simulink model "vehicle_hardware"  (Simulink 7.7)
settings: Solver=ode45  StartTime=0.0  StopTime=10.0  RelTol=1e-3
undefined symbols (not defined in the file): num_robots
libraries: UAVdesign_net x20
settings Model: Creator=Emanuel  LastModifiedBy=Emanuel
settings DebuggingCC: StrictBusMsg=Warning
settings SFSimCC: SimParseCustomCode=off

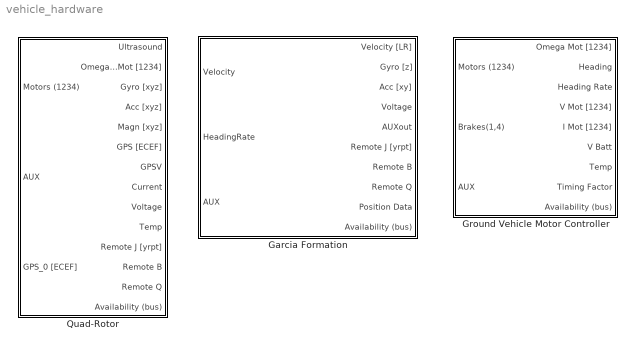
== system vehicle_hardware ==
  Garcia Formation : Subsystem  mask(GarciaFormation){robots_list=[0 1 2 3], sensors_list=[0 1 2 3], use_sensors=off, devicetype=UDP port, com_port='COM4', baud=115200, host_name='192.168.1.10', remote_port=60500, local_port=60500, timeout=1, sample_time=1/20}
      mask prompts: robots_list "List of robots"; sensors_list "List of ultrasound+radio sensors"; use_sensors "Use ultrasound sensors"; devicetype "Device Type"; com_port "COM port (string between commas, e.g. 'COM4')"; baud "Baud Rate"; host_name "Host Name (string between commas, e.g. '192.168.1.10')"; remote_port "Remote UDP port"; local_port "Local UDP port"; timeout "Timeout (sec)"; sample_time "Sample Time"
      mask help:
      | Hardware interface for the Garcia & Track robot formation.
      |
      | If Timeout is zero, the block will not delay the simulation until the data packets arrive. If Timeout is positive and no packet arrives until it elapses, an error will be generated and the simulation will stop.
      mask init:
      | start = 3;
      | a=get_param([gcb '/Generic Comm'], 'MaskStyles');
      | b=get_param(gcb, 'MaskStyles');
      | b{start+1}=a{1};
      | set_param(gcb, 'MaskStyles', b);
      | 
      | a=get_param(gcb, 'MaskValues');
      | b=get_param([gcb '/Generic Comm'], 'MaskValues');
      | b{1}=a{start+1};
      | set_param([gcb '/Generic Comm'], 'MaskValues', b);
      mask StyleString: edit,edit,checkbox,popup(COM port|UDP port),edit,edit,edit,edit,edit,edit,edit
      mask CallbackString:
      | |||start = 3;
      | UAVdesign_net_generic_comm_callback(gcb, 1, start)|||||||
      mask Display:
      | text(0.1, 0.30, ['sensors: ' num2str(sensors_list)])
      | text(0.1, 0.40, ['robots: ' num2str(robots_list)])
      | text(0.1, 0.70, com_port)
      | text(0.1, 0.60, host_name)
  Ground Vehicle Motor Controller : Subsystem  mask(GroundVehicle){com_port='COM4', timeout=1, sample_time=1/100}
      mask prompts: com_port "COM port"; timeout "Timeout (sec)"; sample_time "Sample Time"
      mask help:
      | Hardware interface for the Ground Vehicle Motor Controller.
      |
      | COM port has to be a string including commas, e.g. 'COM4'.
      | If Timeout is zero, the block will not delay the simulation until the data packets arrive. If Timeout is positive and no packet arrives until it elapses, an error will be generated and the simulation will stop.
      mask Display: disp(com_port)
  Quad-Rotor : Subsystem  mask(QuadRotor){devicetype=UDP port, com_port='COM4', baud=115200, host_name='192.168.1.10', remote_port=60500, local_port=60500, timeout=1, sample_time=1/50}
      mask prompts: devicetype "Device Type"; com_port "COM port (string between commas, e.g. 'COM4')"; baud "Baud Rate"; host_name "Host Name (string between commas, e.g. '192.168.1.10')"; remote_port "Remote UDP port"; local_port "Local UDP port"; timeout "Timeout (sec)"; sample_time "Sample Time"
      mask help:
      | Hardware interface for the QuadRotor.
      |
      | COM port has to be a string including commas, e.g. 'COM4'.
      | If Timeout is zero, the block will not delay the simulation until the data packets arrive. If Timeout is positive and no packet arrives until it elapses, an error will be generated and the simulation will stop.
      mask init:
      | start = 0;
      | a=get_param([gcb '/Generic Comm'], 'MaskStyles');
      | b=get_param(gcb, 'MaskStyles');
      | b{start+1}=a{1};
      | set_param(gcb, 'MaskStyles', b);
      | 
      | a=get_param(gcb, 'MaskValues');
      | b=get_param([gcb '/Generic Comm'], 'MaskValues');
      | b{1}=a{start+1};
      | set_param([gcb '/Generic Comm'], 'MaskValues', b);
      mask StyleString: popup(COM port|UDP port),edit,edit,edit,edit,edit,edit,edit
      mask CallbackString:
      | start = 0;
      | UAVdesign_net_generic_comm_callback(gcb, 1, start)|||||||
      mask Display: disp([com_port '\n' host_name])

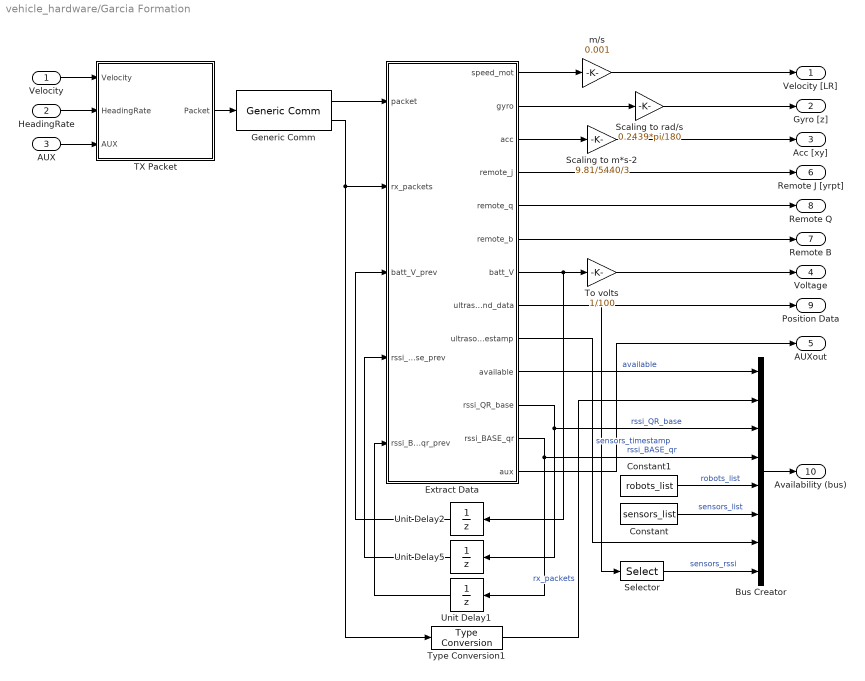
== system vehicle_hardware/Garcia Formation ==
  Velocity : Inport
  HeadingRate : Inport  Port=2
  AUX : Inport  Port=3
  Bus Creator : BusCreator  Inputs=8
  Constant : Constant  Value=sensors_list
  Constant1 : Constant  Value=robots_list
  Extract Data : Stateflow chart  TreatAsAtomicUnit=on
  Generic Comm : UAVdesign_net/Hardware/Generic Comm  SystemSampleTime=-1  devicetype=UDP port  com_port=com_port  baud=baud  host_name=host_name  remote_port=remote_port  local_port=local_port  timeout=timeout  rx_size=(max(robots_list)+1) * 16 + 18 + (4 + 17*8)*use_sensors  handshake=on  sample_time=sample_time
  Scaling to m*s-2 : Gain  Gain=9.81/5440/3
  Scaling to rad/s : Gain  Gain=0.2439*pi/180
  Selector : Selector  InputPortWidth=9*length(sensors_list)*use_sensors + (1-use_sensors)*1  IndexOptions=Index vector (dialog)  Indices=[9*(0:(length(sensors_list)-1)*use_sensors)+9*use_sensors+(1-use_sensors)]  OutputSizes=1
  TX Packet : Subsystem  TreatAsAtomicUnit=on
  To volts : Gain  Gain=1/100
  Type Conversion1 : UAVdesign_net/Hardware/Type Conversion  indim=1  intype=uint32  outdim=1  outtype=double  signextend=off
  Unit Delay1 : UnitDelay  X0=-100*ones(length(robots_list), 1)  SampleTime=-1
  Unit Delay2 : UnitDelay  X0=zeros(length(robots_list), 1)  SampleTime=-1
  Unit Delay5 : UnitDelay  X0=-100*ones(length(robots_list), 1)  SampleTime=-1
  m/s : Gain  Gain=0.001
  Velocity [LR] : Outport
  Gyro [z] : Outport  Port=2
  Acc [xy] : Outport  Port=3
  Voltage : Outport  Port=4
  AUXout : Outport  Port=5
  Remote J [yrpt] : Outport  Port=6
  Remote B : Outport  Port=7
  Remote Q : Outport  Port=8
  Position Data : Outport  Port=9
  Availability (bus) : Outport  Port=10
  wires:
  Extract Data/13(aux) -> AUXout/1
  AUX/1 -> TX Packet/3(AUX)
  Selector/1 -> Bus Creator/8  "sensors_rssi"
  Extract Data/8(ultrasound_data) -> Selector/1, Position Data/1
  Extract Data/9(ultrasound_timestamp) -> Bus Creator/7  "sensors_timestamp"
  Constant/1 -> Bus Creator/6  "sensors_list"
  Constant1/1 -> Bus Creator/5  "robots_list"
  Type Conversion1/1 -> Bus Creator/2  "rx_packets"
  Unit Delay1/1 -> Extract Data/5(rssi_BASE_qr_prev)
  Extract Data/12(rssi_BASE_qr) -> Bus Creator/4, Unit Delay1/1  "rssi_BASE_qr"
  Extract Data/5(remote_q) -> Remote Q/1
  Unit Delay5/1 -> Extract Data/4(rssi_QR_base_prev)
  Extract Data/11(rssi_QR_base) -> Bus Creator/3, Unit Delay5/1  "rssi_QR_base"
  Generic Comm/2 -> Type Conversion1/1, Extract Data/2(rx_packets)
  Unit Delay2/1 -> Extract Data/3(batt_V_prev)
  Generic Comm/1 -> Extract Data/1(packet)
  Extract Data/10(available) -> Bus Creator/1  "available"
  Extract Data/7(batt_V) -> To volts/1, Unit Delay2/1
  Extract Data/6(remote_b) -> Remote B/1
  Extract Data/4(remote_j) -> Remote J [yrpt]/1
  Extract Data/3(acc) -> Scaling to m*s-2/1
  Extract Data/2(gyro) -> Scaling to rad/s/1
  Extract Data/1(speed_mot) -> m/s/1
  Scaling to m*s-2/1 -> Acc [xy]/1
  Scaling to rad/s/1 -> Gyro [z]/1
  m/s/1 -> Velocity [LR]/1
  Bus Creator/1 -> Availability (bus)/1
  To volts/1 -> Voltage/1
  Velocity/1 -> TX Packet/1(Velocity)
  TX Packet/1(Packet) -> Generic Comm/1
  HeadingRate/1 -> TX Packet/2(HeadingRate)

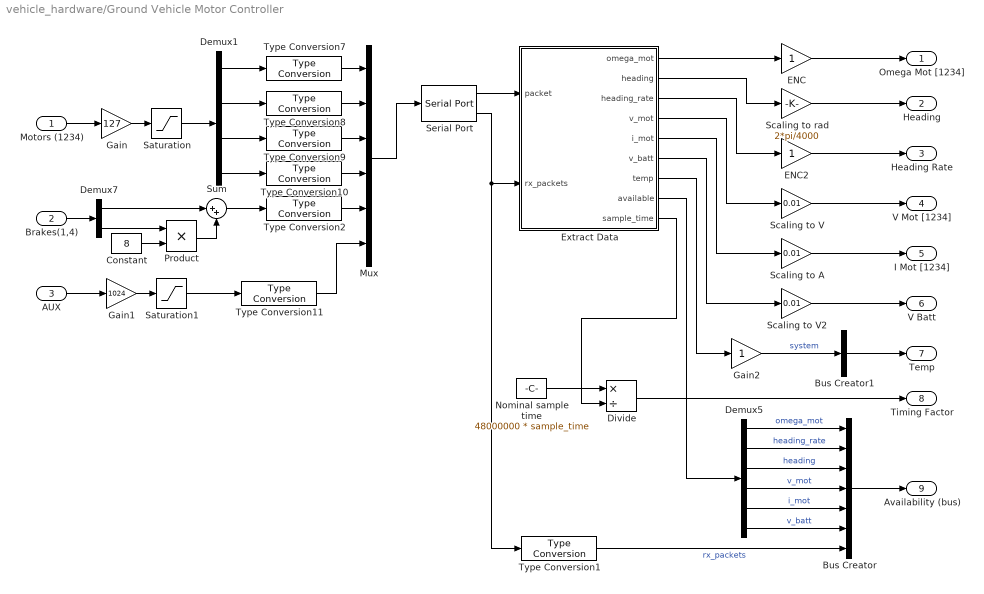
== system vehicle_hardware/Ground Vehicle Motor Controller ==
  Motors (1234) : Inport
  Brakes(1,4) : Inport  Port=2  OutDataTypeStr=boolean  PortDimensions=2
  AUX : Inport  Port=3
  Bus Creator : BusCreator  Inputs=7
  Bus Creator1 : BusCreator  Inputs=1
  Constant : Constant  Value=8
  Demux1 : Demux
  Demux5 : Demux  Outputs=[4 1 1 4 4 1]
  Demux7 : Demux  Outputs=2
  Divide : Product  Inputs=*/
  ENC : Gain
  ENC2 : Gain
  Extract Data : Stateflow chart  TreatAsAtomicUnit=on
  Gain : Gain  Gain=127
  Gain1 : Gain  Gain=1024
  Gain2 : Gain
  Mux : Mux  Inputs=6
  Nominal sample time : Constant  Value=48000000 * sample_time
  Product : Product  RndMeth=Zero
  Saturation : Saturate  UpperLimit=127  LowerLimit=-127
  Saturation1 : Saturate  UpperLimit=1023  LowerLimit=0
  Scaling to A : Gain  Gain=0.01
  Scaling to V : Gain  Gain=0.01
  Scaling to V2 : Gain  Gain=0.01
  Scaling to rad : Gain  Gain=2*pi/4000
  Serial Port : UAVdesign_net/Hardware/Serial Port  port=com_port  baud_rate=115200  timeout=timeout  tx_enable=on  rx_enable=on  receive=56  num_packets_overrun=off  num_packets_received=on  st=sample_time
  Sum : Sum  Inputs=|++  OutDataTypeStr=uint16
  Type Conversion1 : UAVdesign_net/Hardware/Type Conversion  indim=1  intype=uint32  outdim=1  outtype=double  signextend=off
  Type Conversion{7..11} (5 alike) : UAVdesign_net/Hardware/Type Conversion  indim=1  intype=double  outdim=2  outtype=uint8  signextend=off
  Type Conversion2 : UAVdesign_net/Hardware/Type Conversion  indim=1  intype=uint16  outdim=2  outtype=uint8  signextend=off
  Omega Mot [1234] : Outport
  Heading : Outport  Port=2
  Heading Rate : Outport  Port=3
  V Mot [1234] : Outport  Port=4
  I Mot [1234] : Outport  Port=5
  V Batt : Outport  Port=6
  Temp : Outport  Port=7
  Timing Factor : Outport  Port=8
  Availability (bus) : Outport  Port=9
  wires:
  Type Conversion1/1 -> Bus Creator/7  "rx_packets"
  Serial Port/2 -> Extract Data/2(rx_packets), Type Conversion1/1
  Serial Port/1 -> Extract Data/1(packet)
  Extract Data/8(available) -> Demux5/1
  Scaling to V/1 -> V Mot [1234]/1
  Scaling to rad/1 -> Heading/1
  Bus Creator1/1 -> Temp/1
  Bus Creator/1 -> Availability (bus)/1
  Scaling to V2/1 -> V Batt/1
  Gain1/1 -> Saturation1/1
  Saturation1/1 -> Type Conversion11/1
  Saturation/1 -> Demux1/1
  Gain/1 -> Saturation/1
  Motors (1234)/1 -> Gain/1
  Scaling to A/1 -> I Mot [1234]/1
  Mux/1 -> Serial Port/1
  Type Conversion10/1 -> Mux/4
  Type Conversion9/1 -> Mux/3
  Type Conversion8/1 -> Mux/2
  Type Conversion7/1 -> Mux/1
  AUX/1 -> Gain1/1
  Demux1/1 -> Type Conversion7/1
  Demux1/2 -> Type Conversion8/1
  Demux1/3 -> Type Conversion9/1
  Demux1/4 -> Type Conversion10/1
  Brakes(1,4)/1 -> Demux7/1
  Demux7/2 -> Product/1
  Constant/1 -> Product/2
  Sum/1 -> Type Conversion2/1
  Demux7/1 -> Sum/1
  Product/1 -> Sum/2
  Type Conversion11/1 -> Mux/6
  Gain2/1 -> Bus Creator1/1  "system"
  Demux5/1 -> Bus Creator/1  "omega_mot"
  Extract Data/1(omega_mot) -> ENC/1
  Extract Data/2(heading) -> Scaling to rad/1
  Extract Data/4(v_mot) -> Scaling to V/1
  Extract Data/5(i_mot) -> Scaling to A/1
  Extract Data/6(v_batt) -> Scaling to V2/1
  Extract Data/7(temp) -> Gain2/1
  Type Conversion2/1 -> Mux/5
  Extract Data/9(sample_time) -> Divide/2
  Divide/1 -> Timing Factor/1
  Nominal sample time/1 -> Divide/1
  ENC/1 -> Omega Mot [1234]/1
  Demux5/6 -> Bus Creator/6  "v_batt"
  Demux5/5 -> Bus Creator/5  "i_mot"
  Demux5/4 -> Bus Creator/4  "v_mot"
  Demux5/3 -> Bus Creator/3  "heading"
  Demux5/2 -> Bus Creator/2  "heading_rate"
  ENC2/1 -> Heading Rate/1
  Extract Data/3(heading_rate) -> ENC2/1

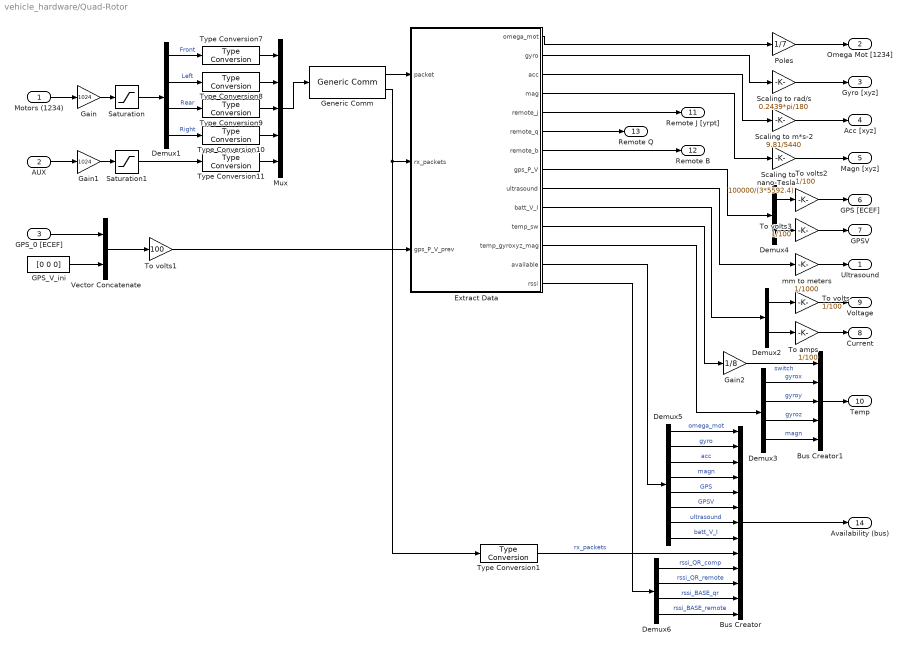
== system vehicle_hardware/Quad-Rotor ==
  Motors (1234) : Inport
  AUX : Inport  Port=2
  GPS_0 [ECEF] : Inport  Port=3
  Bus Creator : BusCreator  Inputs=13
  Bus Creator1 : BusCreator  Inputs=5
  Demux1 : Demux
  Demux2 : Demux  Outputs=2
  Demux3 : Demux
  Demux4 : Demux  Outputs=2
  Demux5 : Demux  Outputs=[4 3 3 3 3 3 1 1]
  Demux6 : Demux
  Extract Data : Stateflow chart  TreatAsAtomicUnit=on
  GPS_V_ini : Constant  Value=[0 0 0]
  Gain : Gain  Gain=1024
  Gain1 : Gain  Gain=1024
  Gain2 : Gain  Gain=1/8
  Generic Comm : UAVdesign_net/Hardware/Generic Comm  SystemSampleTime=-1  devicetype=UDP port  com_port=com_port  baud=baud  host_name=host_name  remote_port=remote_port  local_port=local_port  timeout=timeout  rx_size=54  handshake=on  sample_time=sample_time
  Mux : Mux  Inputs=5
  Poles : Gain  Gain=1/7
  Saturation : Saturate  UpperLimit=1023  LowerLimit=0
  Saturation1 : Saturate  UpperLimit=1023  LowerLimit=0
  Scaling to m*s-2 : Gain  Gain=9.81/5440
  Scaling to nano-Tesla : Gain  Gain=100000/(3*5592.4)
  Scaling to rad/s : Gain  Gain=0.2439*pi/180
  To amps : Gain  Gain=1/100
  To volts : Gain  Gain=1/100
  To volts1 : Gain  Gain=100
  To volts2 : Gain  Gain=1/100
  To volts3 : Gain  Gain=1/100
  Type Conversion1 : UAVdesign_net/Hardware/Type Conversion  indim=1  intype=uint32  outdim=1  outtype=double  signextend=off
  Type Conversion{7..11} (5 alike) : UAVdesign_net/Hardware/Type Conversion  indim=1  intype=double  outdim=2  outtype=uint8  signextend=off
  Vector Concatenate : Concatenate  Mode=Vector
  mm to meters : Gain  Gain=1/1000
  Ultrasound : Outport
  Omega Mot [1234] : Outport  Port=2
  Gyro [xyz] : Outport  Port=3
  Acc [xyz] : Outport  Port=4
  Magn [xyz] : Outport  Port=5
  GPS [ECEF] : Outport  Port=6
  GPSV : Outport  Port=7
  Current : Outport  Port=8
  Voltage : Outport  Port=9
  Temp : Outport  Port=10
  Remote J [yrpt] : Outport  Port=11
  Remote B : Outport  Port=12
  Remote Q : Outport  Port=13
  Availability (bus) : Outport  Port=14
  wires:
  Extract Data/6(remote_q) -> Remote Q/1
  Type Conversion1/1 -> Bus Creator/9  "rx_packets"
  Demux6/4 -> Bus Creator/13  "rssi_BASE_remote"
  Demux6/3 -> Bus Creator/12  "rssi_BASE_qr"
  Demux6/2 -> Bus Creator/11  "rssi_QR_remote"
  Demux6/1 -> Bus Creator/10  "rssi_QR_comp"
  Extract Data/14(rssi) -> Demux6/1
  Generic Comm/2 -> Type Conversion1/1, Extract Data/2(rx_packets)
  GPS_V_ini/1 -> Vector Concatenate/2
  GPS_0 [ECEF]/1 -> Vector Concatenate/1
  Vector Concatenate/1 -> To volts1/1
  To volts1/1 -> Extract Data/3(gps_P_V_prev)
  Generic Comm/1 -> Extract Data/1(packet)
  Extract Data/13(available) -> Demux5/1
  Demux5/8 -> Bus Creator/8  "batt_V_I"
  Demux5/7 -> Bus Creator/7  "ultrasound"
  Demux5/6 -> Bus Creator/6  "GPSV"
  Demux5/5 -> Bus Creator/5  "GPS"
  Demux5/4 -> Bus Creator/4  "magn"
  Demux5/3 -> Bus Creator/3  "acc"
  Demux5/2 -> Bus Creator/2  "gyro"
  Demux5/1 -> Bus Creator/1  "omega_mot"
  Extract Data/12(temp_gyroxyz_mag) -> Demux3/1
  Extract Data/11(temp_sw) -> Gain2/1
  Extract Data/10(batt_V_I) -> Demux2/1
  Extract Data/9(ultrasound) -> mm to meters/1
  Extract Data/7(remote_b) -> Remote B/1
  Extract Data/5(remote_j) -> Remote J [yrpt]/1
  Extract Data/4(mag) -> Scaling to nano-Tesla/1
  Extract Data/3(acc) -> Scaling to m*s-2/1
  Extract Data/2(gyro) -> Scaling to rad/s/1
  Extract Data/1(omega_mot) -> Poles/1
  Extract Data/8(gps_P_V) -> Demux4/1
  Demux4/2 -> To volts3/1
  Demux4/1 -> To volts2/1
  To volts3/1 -> GPSV/1
  To volts2/1 -> GPS [ECEF]/1
  Scaling to m*s-2/1 -> Acc [xyz]/1
  Scaling to rad/s/1 -> Gyro [xyz]/1
  Poles/1 -> Omega Mot [1234]/1
  Demux2/2 -> To amps/1
  Demux2/1 -> To volts/1
  Demux3/4 -> Bus Creator1/5  "magn"
  Demux3/3 -> Bus Creator1/4  "gyroz"
  Demux3/2 -> Bus Creator1/3  "gyroy"
  Demux3/1 -> Bus Creator1/2  "gyrox"
  Gain2/1 -> Bus Creator1/1  "switch"
  Bus Creator1/1 -> Temp/1
  Bus Creator/1 -> Availability (bus)/1
  To volts/1 -> Voltage/1
  To amps/1 -> Current/1
  mm to meters/1 -> Ultrasound/1
  Gain1/1 -> Saturation1/1
  Saturation1/1 -> Type Conversion11/1
  Saturation/1 -> Demux1/1
  Gain/1 -> Saturation/1
  Demux1/3 -> Type Conversion9/1  "Rear"
  Demux1/2 -> Type Conversion8/1  "Left"
  Demux1/4 -> Type Conversion10/1  "Right"
  Demux1/1 -> Type Conversion7/1  "Front"
  Motors (1234)/1 -> Gain/1
  Scaling to nano-Tesla/1 -> Magn [xyz]/1
  Mux/1 -> Generic Comm/1
  Type Conversion11/1 -> Mux/5
  Type Conversion10/1 -> Mux/4
  Type Conversion9/1 -> Mux/3
  Type Conversion8/1 -> Mux/2
  Type Conversion7/1 -> Mux/1
  AUX/1 -> Gain1/1

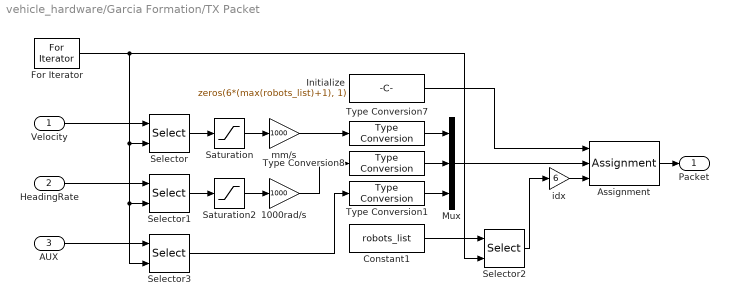
== system vehicle_hardware/Garcia Formation/TX Packet ==
  Velocity : Inport
  HeadingRate : Inport  Port=2
  AUX : Inport  Port=3  OutDataTypeStr=uint16
  1000rad/s : Gain  Gain=1000
  Assignment : Assignment  IndexMode=Zero-based  IndexOptions=Starting index (port)  Indices=1  OutputSizes=num_robots * 4
  Constant1 : Constant  Value=robots_list  OutDataTypeStr=uint32
  For Iterator : ForIterator  IterationLimit=length(robots_list)  IndexMode=Zero-based
  Initialize : Constant  Value=zeros(6*(max(robots_list)+1), 1)  OutDataTypeStr=uint8
  Mux : Mux  Inputs=3
  Saturation : Saturate  UpperLimit=1  LowerLimit=-1
  Saturation2 : Saturate  UpperLimit=2*pi  LowerLimit=-2*pi
  Selector{,1..3} (4 alike) : Selector  IndexMode=Zero-based  InputPortWidth=length(robots_list)  IndexOptions=Starting index (port)  Indices=[1 3]  OutputSizes=1
  Type Conversion1 : UAVdesign_net/Hardware/Type Conversion  indim=1  intype=uint16  outdim=2  outtype=uint8  signextend=off
  Type Conversion7 : UAVdesign_net/Hardware/Type Conversion  indim=1  intype=double  outdim=2  outtype=uint8  signextend=off
  Type Conversion8 : UAVdesign_net/Hardware/Type Conversion  indim=1  intype=double  outdim=2  outtype=uint8  signextend=off
  idx : Gain  Gain=6  ParamDataTypeStr=int32  OutDataTypeStr=int32
  mm/s : Gain  Gain=1000
  Packet : Outport
  wires:
  Type Conversion1/1 -> Mux/3
  Selector3/1 -> Type Conversion1/1
  AUX/1 -> Selector3/1
  Selector2/1 -> idx/1
  idx/1 -> Assignment/3
  Constant1/1 -> Selector2/1
  Initialize/1 -> Assignment/1
  Mux/1 -> Assignment/2
  Assignment/1 -> Packet/1
  For Iterator/1 -> Selector2/2, Selector3/2, Selector1/2, Selector/2
  HeadingRate/1 -> Selector1/1
  Selector1/1 -> Saturation2/1
  Selector/1 -> Saturation/1
  Velocity/1 -> Selector/1
  Type Conversion8/1 -> Mux/2
  Type Conversion7/1 -> Mux/1
  Saturation/1 -> mm/s/1
  Saturation2/1 -> 1000rad/s/1
  mm/s/1 -> Type Conversion7/1
  1000rad/s/1 -> Type Conversion8/1

== matlab function Garcia Formation/Extract Data ==
  data: packet input uint8; rx_packets input uint32; speed_mot output double; gyro output double; acc output double; remote_j output double size=4; remote_q output double size=4; remote_b output uint16 size=1; batt_V output double; ultrasound_data output double; ultrasound_timestamp output double; available output boolean; batt_V_prev input double; rssi_QR_base output double; rssi_QR_base_prev input double; robots_list parameter double; rssi_BASE_qr_prev input double; rssi_BASE_qr output double; sensors_list parameter double; use_sensors parameter double; aux output uint8
function [speed_mot,gyro, acc, remote_j, remote_q, remote_b, batt_V, ultrasound_data, ultrasound_timestamp, available, rssi_QR_base, rssi_BASE_qr, aux] = unpack(packet, rx_packets, batt_V_prev, rssi_QR_base_prev, robots_list, rssi_BASE_qr_prev, sensors_list, use_sensors)

robot_packet_size = 16;
num_robots = length(robots_list);
if num_robots < 1 || num_robots > 8
    error('A mimimum of 1 and a maximum of 8 robots can be used.');
end
if min(robots_list) < 0 || max(robots_list) > 7
   error('The robot identifiers must be between 0 and 7.'); 
end

speed_mot =         zeros(2*num_robots, 1);
gyro      =         zeros(  num_robots, 1);
acc       =         zeros(2*num_robots, 1);
aux       =         zeros(num_robots, 1, 'uint8');
available = logical(zeros(  num_robots, 1));

batt_V       = batt_V_prev;
rssi_QR_base = rssi_QR_base_prev;
rssi_BASE_qr = rssi_BASE_qr_prev;

for i=1:num_robots
    
    start = robots_list(i)*robot_packet_size;       % start of packet for the current robot (zero based)
    
    if rx_packets > 0
        MUX = uint8(packet(start+10));
    else
        MUX = uint8(0);
    end

    if MUX
        available(i) = logical(1);
    else
        available(i) = logical(0);
        rssi_QR_base(i) = -100;
        rssi_BASE_qr(i) = -100;
    end

    switch MUX
        case 4
            batt_V(i) = double(typecast(packet(start+(7:8)), 'uint16'));
        case 8
            rssi_QR_base(i) = -double(typecast(packet(start+5), 'uint8'));
            rssi_BASE_qr(i) = -double(typecast(packet(start+7), 'uint8'));
    end

    % speed_mot is actually the linear velocity in mm/sec for each wheel
    speed_mot(2*(i-1)+(1:2)) = double(typecast(packet(start+(11:14)), 'int16'));

    % the gyroscope data has to be scaled externally to rad/sec
    gyro(i) = double(typecast(packet(start+(15:16)), 'int16'));

    % the acceleration data has to be scaled externally to m/sec^2
    acc(2*(i-1)+(1:2)) = double(typecast(packet(start+(1:4)), 'int16'));
    
    % the AUX channels
    aux(i) = uint8(packet(start+9));
end
start = (max(robots_list)+1)*robot_packet_size;

% remote control data
remote_j = [double(typecast(packet(start+(1:6)), 'int16')); double(typecast(packet(start+(7:8)), 'uint16'))];
remote_j = remote_j .* [1/512; 1/512; 1/512; 1/1024] - [1; 1; 1; 0];
remote_b = typecast(packet(start+(9:10)), 'uint16');
remote_q = double(typecast(packet(start+(11:18)), 'int16'));
remote_q = remote_q / 2^15;
start = start + 18;

% ultrasound data
if use_sensors
    num_sensors = length(sensors_list);
    ultrasound_data = zeros(9*num_sensors, 1);
    sensor_packet_size = 17;

    if num_sensors < 1 || num_sensors > 8
        error('A mimimum of 1 and a maximum of 8 sensors can be used.');
    end
    if min(sensors_list) < 0 || max(sensors_list) > 7
       error('The robot identifiers must be between 0 and 7.'); 
    end

    ultrasound_timestamp = double(typecast(packet(start+(1:4)), 'uint32')) * 6.4;
    for i=1:num_sensors
        start2 = start + 4 + sensors_list(i)*sensor_packet_size;       % start of packet for the current robot (zero based)
        ultrasound_data(9*(i-1)+1) = double(typecast(packet(start2+(1:2)), 'uint16')) * 0.005;
        ultrasound_data(9*(i-1)+2) = double(typecast(packet(start2+(3:4)), 'uint16')) * 0.01;
        ultrasound_data(9*(i-1)+3) = double(typecast(packet(start2+(5:8)), 'uint32')) * 6.4;
        ultrasound_data(9*(i-1)+4) = double(typecast(packet(start2+(9:12)),'uint32')) * 6.4;
        ultrasound_data(9*(i-1)+5) = double(typecast(packet(start2+13),    'uint8' ));
        ultrasound_data(9*(i-1)+6) = double(typecast(packet(start2+14),    'uint8' ));
        ultrasound_data(9*(i-1)+7) = double(typecast(packet(start2+15),    'uint8' ));
        ultrasound_data(9*(i-1)+8) = double(typecast(packet(start2+16),    'uint8' ));
        ultrasound_data(9*(i-1)+9) = double(typecast(packet(start2+17),    'uint8' ));
    end
else
    ultrasound_data = 0;
    ultrasound_timestamp = 0;
end

== matlab function Ground Vehicle Motor Controller/Extract Data ==
  data: packet input uint8; rx_packets input uint32; omega_mot output double size=4; heading output double size=1; heading_rate output double size=1; v_mot output double size=4; i_mot output double size=4; v_batt output double size=1; temp output double size=1; available output boolean size=15; sample_time output double size=1
function [omega_mot, heading, heading_rate, v_mot, i_mot, v_batt, temp, available, sample_time] = unpack(packet, rx_packets)

if rx_packets > 0
    MUX = uint8(packet(10));
else
    MUX = uint8(0);
end

% available: omega_mot heading v_mot i_mot v_batt
if MUX
    available = logical([1 1 1 1 1   1   1 1 1 1   1 1 1 1   1]');
else
    available = logical([0 0 0 0 0   0   0 0 0 0   0 0 0 0   0]');
end

v_batt = double(typecast(packet(7:8), 'uint16'));
temp   = double(typecast(packet(11:12), 'int16' ));

% omega_mot: multiply with (1/N_encoder_counts) externally
% N_encoder_counts is the number of lines (not the number of events = 4 x lines)
period_mot = double(typecast(packet(13:28), 'int32'));
omega_mot = zeros(4,1);
for i=1:4
    if (period_mot(i)<=-0.5) || (period_mot(i) >= 0.5)
        omega_mot(i) = 2*pi * 10^6 *48 / period_mot(i);
    end
end

% heading_rate: multiply with (1/N_encoder_counts) externally
% N_encoder_counts is the number of lines (not the number of events = 4 x lines)
period_heading = double(typecast(packet(29:32), 'int32'));
heading_rate = 0;
if (period_heading<=-1) || (period_heading >= 1)
    heading_rate = 2*pi * 10^6 *48 / period_heading;
end

heading   = double(typecast(packet(33:36), 'int32'));
v_mot     = double(typecast(packet(37:44), 'int16'));
i_mot     = double(typecast(packet(45:52), 'int16'));

% sample time: represents 48 x (time in microseconds) that goes between two sample points
sample_time = double(typecast(packet(53:56), 'uint32'));
if sample_time == 0
    sample_time = 1;
end

== matlab function Quad-Rotor/Extract Data ==
  data: packet input uint8; rx_packets input uint32; gps_P_V_prev input double size=6; omega_mot output double size=4; gyro output double size=3; acc output double size=3; mag output double size=3; remote_j output double size=4; remote_q output double size=4; remote_b output uint16 size=1; gps_P_V output double size=6; ultrasound output double size=1; batt_V_I output double size=2; temp_sw output double size=1; temp_gyroxyz_mag output double size=4; available output boolean size=21; rssi output double
function [omega_mot,gyro, acc, mag, remote_j, remote_q, remote_b, gps_P_V, ultrasound, batt_V_I, temp_sw, temp_gyroxyz_mag, available, rssi] = unpack(packet, rx_packets, gps_P_V_prev)

persistent prev_data

if isempty(prev_data)
    prev_data = [gps_P_V_prev; 0; 0; 0; 0; 0; 0; 0; 0; -100; -100; -100; -100];
end

gps_P_V  = prev_data(1:6);
ultrasound = prev_data(7);
batt_V_I = prev_data(8:9);
temp_sw = prev_data(10);
temp_gyroxyz_mag = prev_data(11:14);
rssi = prev_data(15:18);

if rx_packets > 0
    MUX = uint8(packet(10));
else
    MUX = uint8(0);
end

% available: omega_mot  gyro  acc  magn  GPS  GPSV  ultrasound  current_voltage
if MUX
    available = logical([1 1 1 1   1 1 1   1 1 1   1 1 1   0 0 0   0 0 0   0  0]');
else
    available = logical([0 0 0 0   0 0 0   0 0 0   0 0 0   0 0 0   0 0 0   0  0]');
    rssi = [-100 -100 -100 -100]';
end

if bitand(MUX, 128)
    ultrasound = double(typecast(packet(1:4), 'uint32'));
    available(20) = true;
end

MUX = uint8(bitand(MUX, 127));

switch MUX
    case 1
        gps_P_V(1) = double(typecast(packet(1:4), 'int32'));
        gps_P_V(2) = double(typecast(packet(5:8), 'int32'));
        available(14:15) = logical([1; 1]);
    case 2
        gps_P_V(3) = double(typecast(packet(1:4), 'int32'));
        a = uint8(0);
        if bitand(packet(7), 128)
            a = uint8(255);
        end
        gps_P_V(6) = double(typecast([packet(5:7); a], 'int32'));
        available([16 19]) = logical([1; 1]);
    case 3
        a = uint8(0);
        if bitand(packet(3), 128)
            a = uint8(255);
        end
        gps_P_V(4) = double(typecast([packet(1:3); a], 'int32'));
        a = uint8(0);
        if bitand(packet(7), 128)
            a = uint8(255);
        end
        gps_P_V(5) = double(typecast([packet(5:7); a], 'int32'));
        available(17:18) = logical([1; 1]);
    case 4
        batt_V_I(1) = double(typecast(packet(7:8), 'uint16'));
        batt_V_I(2) = double(typecast(packet(5:6), 'uint16'));
        available(21) = true;
    case 5
        temp_sw = double(typecast(packet(5:6), 'int16'));
    case 6
        temp_gyroxyz_mag(1:2) = double(typecast(packet(5:8), 'uint16'));
    case 7
        temp_gyroxyz_mag(3:4) = double(typecast(packet(5:8), 'uint16'));
    case 8
        rssi = -double(typecast(packet(5:8), 'uint8'));
end

% omega_mot has to be divided by half the number of poles externally
period_mot = double(typecast(packet(11:18), 'uint16'));
omega_mot = zeros(4,1);
for i=1:4
    if period_mot(i)
        omega_mot(i) = 2*pi * 10^6 / period_mot(i);
    end
end

% the gyroscope data has to be scaled externally to rad/sec
gyro = double(typecast(packet(19:24), 'int16'));

% the acceleration data has to be scaled externally to m/sec^2
acc = double(typecast(packet(25:30), 'int16'));

% the magnetometer data has to be scaled externally to nT
mag = double(typecast(packet(31:36), 'int16'));

% remote control data
remote_j = [double(typecast(packet(37:42), 'int16')); double(typecast(packet(43:44), 'uint16'))];
remote_j = remote_j .* [1/512; 1/512; 1/512; 1/1024] - [1; 1; 1; 0];
remote_b = typecast(packet(45:46), 'uint16');
remote_q = double(typecast(packet(47:54), 'int16'));
remote_q = remote_q / 2^15;
if remote_q' * remote_q < 0.5
    remote_q = [1; 0; 0; 0];
end

% store current values
prev_data = [gps_P_V; ultrasound; batt_V_I; temp_sw; temp_gyroxyz_mag; rssi];
